simulink model "LQR"  (R2020a)
settings: Solver=ode45  StartTime=0.0  StopTime=10.0  RelTol=1e-3  EnableMultiTasking=on
values from neighbouring files (symbols this model uses):
  A = [0 0 0 0 ... (first row only)    [StateSpaceMatrices.m]    (also in robotFoR.m = [cosd(theta), sind(theta), 0; shit.m = [1 -0.2094 1)
  B = [1/m, 1/m, 0, 0 ... (first row only)    [StateSpaceMatrices.m]    (also in barrier.m = sym(zeros(N,1)); shit.m = [1 0)
  Q = eye(m)    [Decentralised2D.m]    (also in shit.m = diag([5.5 5.5 216.5]))
  R = eye(m)    [Decentralised2D.m]    (also in shit.m = diag([1 1]))
undefined symbols (not defined in the file or in its folder): X0
libraries: dspinverses x1
settings Model: Creator=gkavuran  LastModifiedBy=javier
settings DataIOCC: LimitDataPoints=on  SaveFormat=Array  ReturnWorkspaceOutputs=off
settings OptimizationCC: LifeSpan=inf
settings DebuggingCC: SolverPrmCheckMsg=warning  SFUnexpectedBacktrackingDiag=warning  SFNoUnconditionalDefaultTransitionDiag=warning  SFExecutionAtInitializationDiag=none  ArithmeticOperatorsInVariantConditions=warning
settings HardwareCC: ProdBitPerPointer=32  ProdBitPerSizeT=32  ProdBitPerPtrDiffT=32  ProdLargestAtomicFloat=None  ProdIntDivRoundTo=Undefined  ProdEndianess=Unspecified  ProdWordSize=32  ProdHWDeviceType=32-bit Generic
settings ModelReferenceCC: PropagateSignalLabelsOutOfModel=off
settings SFSimCC: SimUseLocalCustomCode=off  CustomCodeUndefinedFunction=UseInterfaceOnly
settings RTWCC: RTWUseLocalCustomCode=off
settings CodeAppCC: StateflowObjectComments=on
settings GRTTargetCC: TargetLangStandard=C89/C90 (ANSI)
settings ConfigComp: CovMetricSettings=dw  CovHtmlReporting=on  CovSaveCumulativeToWorkspaceVar=on  CovSaveSingleToWorkspaceVar=on  CovExternalEMLEnable=off  CovSFcnEnable=off

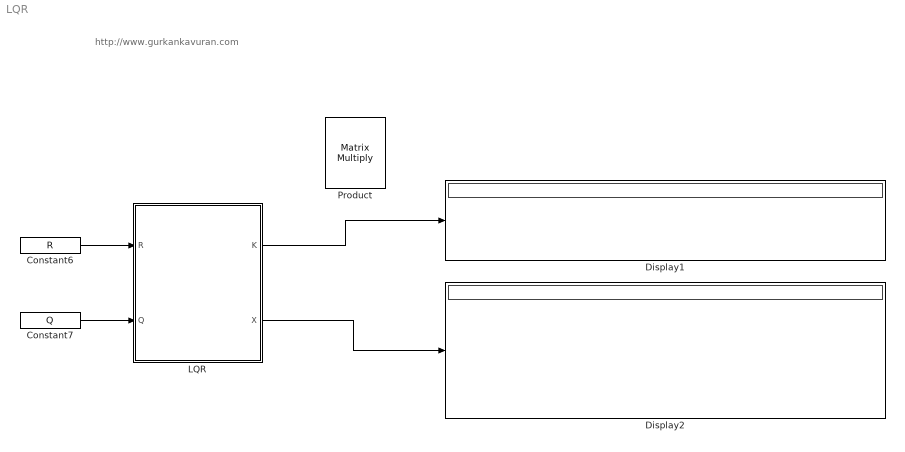
== system LQR ==
  note: http://www.gurkankavuran.com
  Constant6 : Constant  Value=R
  Constant7 : Constant  Value=Q
  Display1 : Display
  Display2 : Display
  LQR : Subsystem  Description=|  TreatAsAtomicUnit=on  mask(LQR with Algebric Riccati Equation){A=A, B=B, X0=X0}
      | LQR Block
      | 
      | by Gurkan KAVURAN
      | gurkankavuran@gmail.com
      mask prompts: A "A (System Matrix)"; B "B (System Matrix)"; X0 "Xo (Initial Values of States)"
      mask help:
      | It is easy to optimize Q and R matrices with online process.
      | Please see the help file to define the block parameters.
      mask Help:
      | Parameters Example:
      | 
      | Q = diag([500 1 1 0 1 1] );
      | R = 1*diag([0.01 0.01 0.01 0.01]);
      | X0=[0 0 0 0 0 0;0 0 0 0 0 0;0 0 0 0 0 0;0 0 0 0 0 0;0 0 0 0 0 0;0 0 0 0 0 0];
      | 
      | "Matrix multiply" block is recommended to use in state feedback control mechanism.
      | 
      | 
      | http://www.gurkankavuran.com
      mask Display:
      | disp('LQR')
      | port_label('input', 1, 'R')
      | port_label('input', 2, 'Q')
      | port_label('output', 1, 'K')
      | port_label('output', 2, 'X')
  Product : Product  Multiplication=Matrix(*)
  wires:
  LQR/1(K) -> Display1/1
  Constant6/1 -> LQR/1(R)
  Constant7/1 -> LQR/2(Q)
  LQR/2(X) -> Display2/1

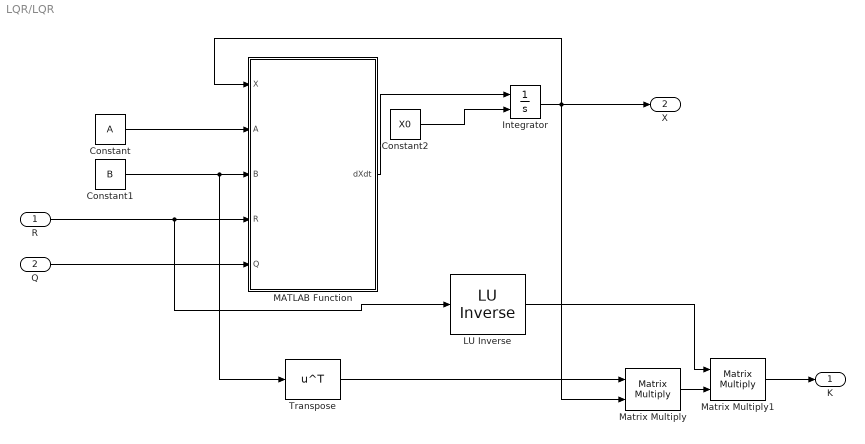
== system LQR/LQR ==
  R : Inport
  Q : Inport  Port=2
  " LU Inverse" : dspinverses/ LU Inverse
  Constant : Constant  Value=A
  Constant1 : Constant  Value=B
  Constant2 : Constant  Value=X0
  Integrator : Integrator  InitialConditionSource=external  InitialCondition=[1 1 1 1 1 1 1 1 1 1 1 1 1 1 1 1 1 1 1 1 1 1 1 1 1 1 1 1 1 1 1 1 1 1 1 1]
  MATLAB Function : MATLAB Function  TreatAsAtomicUnit=on
  Matrix Multiply : Product  Multiplication=Matrix(*)
  Matrix Multiply1 : Product  Multiplication=Matrix(*)
  Transpose : Math  Operator=transpose  SaturateOnIntegerOverflow=on
  K : Outport
  X : Outport  Port=2
  wires:
  Matrix Multiply1/1 -> K/1
  Constant/1 -> MATLAB Function/2(A)
  Constant1/1 -> Transpose/1, MATLAB Function/3(B)
  " LU Inverse"/1 -> Matrix Multiply1/1
  Constant2/1 -> Integrator/2
  Matrix Multiply/1 -> Matrix Multiply1/2
  Transpose/1 -> Matrix Multiply/1
  MATLAB Function/1(dXdt) -> Integrator/1
  Integrator/1 -> X/1, Matrix Multiply/2, MATLAB Function/1(X)
  Q/1 -> MATLAB Function/5(Q)
  R/1 -> " LU Inverse"/1, MATLAB Function/4(R)

== matlab function LQR/MATLAB Function ==
  data: dXdt output; X input; A input; B input; R input; Q input
function dXdt  = mRiccati(X, A, B,R,Q)
% r1=randi([1 1000]);
% r2=randi([1 1000]);
% r3=randi([1 1000]);
% r4=randi([1 1000]);
% r5=randi([1 1000]);
% r6=randi([1 1000]);
% Q = diag([r1 r2 r3 r4 r5 r6] );
% R = 1*diag([1 1 1 1]);
% X = reshape(X, size(A)); %Convert from "n^2"-by-1 to "n"-by-"n"
dXdt = A.'*X + X*A - (X*B)*inv(R)*(B.'*X) + Q; %Determine derivative
% dXdtS= dXdt(:); %Convert from "n"-by-"n" to "n^2"-by-1,algebraic Riccati equation (ARE)
